simulink model "lqr_2dof_nonlinear_force"  (R2017a)
settings: Solver=ode45  StartTime=0.0  StopTime=50  RelTol=1e-3
undefined symbols (not defined in the file): f, g, GoalPos, K, l, m_p
settings Model: Creator=sansh  LastModifiedBy=rj2318

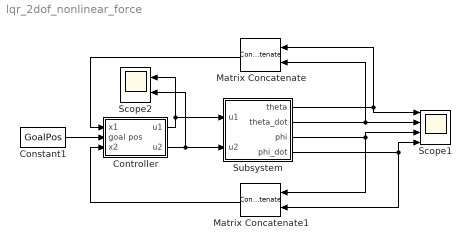
== system lqr_2dof_nonlinear_force ==
  Constant1 : Constant  Value=GoalPos
  Controller : Subsystem
  Matrix Concatenate : Concatenate  Mode=Multidimensional array  ConcatenateDimension=2
  Matrix Concatenate1 : Concatenate  Mode=Multidimensional array  ConcatenateDimension=2
  Scope1 : Scope  NumInputPorts=4
  Scope2 : Scope  NumInputPorts=2
  Subsystem : Subsystem
  wires:
  Subsystem/4(phi_dot) -> Scope1/4, Matrix Concatenate1/2
  Subsystem/3(phi) -> Matrix Concatenate1/1, Scope1/3
  Controller/2(u2) -> Scope2/2, Subsystem/2(u2)
  Constant1/1 -> Controller/2(goal pos)
  Controller/1(u1) -> Scope2/1, Subsystem/1(u1)
  Subsystem/1(theta) -> Matrix Concatenate/1, Scope1/1
  Subsystem/2(theta_dot) -> Matrix Concatenate/2, Scope1/2
  Matrix Concatenate1/1 -> Controller/3(x2)
  Matrix Concatenate/1 -> Controller/1(x1)

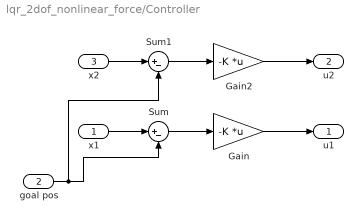
== system lqr_2dof_nonlinear_force/Controller ==
  x1 : Inport
  goal pos : Inport  Port=2
  x2 : Inport  Port=3
  Gain : Gain  Gain=-K  Multiplication=Matrix(K*u)
  Gain2 : Gain  Gain=-K  Multiplication=Matrix(K*u)
  Sum : Sum  Inputs=|+-
  Sum1 : Sum  Inputs=|+-
  u1 : Outport
  u2 : Outport  Port=2
  wires:
  x1/1 -> Sum/1
  Gain/1 -> u1/1
  Sum/1 -> Gain/1
  Gain2/1 -> u2/1
  Sum1/1 -> Gain2/1
  goal pos/1 -> Sum1/2, Sum/2
  x2/1 -> Sum1/1

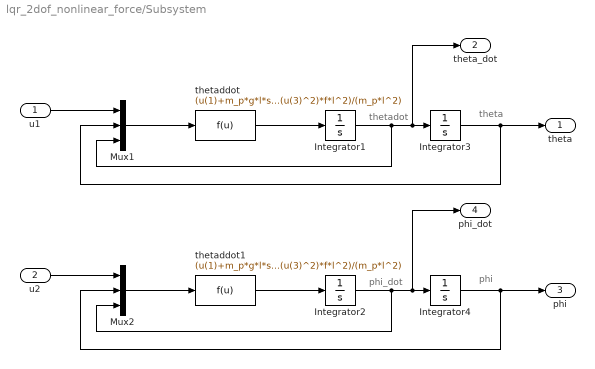
== system lqr_2dof_nonlinear_force/Subsystem ==
  note: theta
  note: thetadot
  note: phi
  note: phi_dot
  u1 : Inport
  u2 : Inport  Port=2
  Integrator1 : Integrator  ContinuousStateAttributes='thetadot'
  Integrator2 : Integrator  ContinuousStateAttributes='thetadot'
  Integrator3 : Integrator  InitialCondition=0.1  ContinuousStateAttributes='theta'
  Integrator4 : Integrator  InitialCondition=0.1  ContinuousStateAttributes='theta'
  Mux1 : Mux  Inputs=3
  Mux2 : Mux  Inputs=3
  thetaddot : Fcn  Expr=(u(1)+m_p*g*l*sin(u(2))-(u(3)^2)*f*l^2)/(m_p*l^2)
  thetaddot1 : Fcn  Expr=(u(1)+m_p*g*l*sin(u(2))-(u(3)^2)*f*l^2)/(m_p*l^2)
  theta : Outport
  theta_dot : Outport  Port=2
  phi : Outport  Port=3
  phi_dot : Outport  Port=4
  wires:
  Mux1/1 -> thetaddot/1
  thetaddot/1 -> Integrator1/1
  Integrator1/1 -> Mux1/3, theta_dot/1, Integrator3/1
  Integrator3/1 -> Mux1/2, theta/1
  u1/1 -> Mux1/1
  Integrator4/1 -> Mux2/2, phi/1
  thetaddot1/1 -> Integrator2/1
  u2/1 -> Mux2/1
  Mux2/1 -> thetaddot1/1
  Integrator2/1 -> Mux2/3, phi_dot/1, Integrator4/1
